simulink model "basic"  (R2018a)
settings: Solver=FixedStepAuto  StartTime=0.0  StopTime=inf  FixedStep=0.005  RelTol=1e-3  EnableMultiTasking=on
libraries: arduinolib x3, simulink x3
settings Model: SimulationMode=external  ExtModeTrigDuration=2  Creator=adiravishankara  LastModifiedBy=adiravishankara
settings SolverCC: AutoInsertRateTranBlk=on
settings OptimizationCC: EnhancedBackFolding=on  PassReuseOutputArgsAs=Individual arguments  MaxStackSize=64  OptimizeBlockOrder=speed  DifferentSizesBufferReuse=on  OptimizationCustomize=off
settings DebuggingCC: ParameterTunabilityLossMsg=error
settings HardwareCC: ProdBitPerPointer=32  ProdBitPerSizeT=32  ProdBitPerPtrDiffT=32  ProdLargestAtomicInteger=Long  ProdLargestAtomicFloat=Double  ProdWordSize=32  ProdHWDeviceType=ARM Compatible->ARM Cortex  UseEmbeddedCoderFeatures=off
settings SFSimCC: MATLABDynamicMemAlloc=off
settings RTWCC: SystemTargetFile=ert.tlc  HardwareBoard=Arduino Due  TLCOptions=-aInlineSetEventsForThisBaseRateFcn=TLC_FALSE -aSuppressMultiTaskScheduler=TLC_FALSE -aRateBasedStepFcn=1  TemplateMakefile=ert_default_tmf  GenerateReport=on  Toolchain=Arduino ARM  BuildConfiguration=Faster Runs  IncludeHyperlinkInReport=on  LaunchReport=on  GenerateTraceInfo=on  GenerateTraceReport=on  GenerateTraceReportSl=on  GenerateTraceReportSf=on  GenerateTraceReportEml=on
settings CodeAppCC: ForceParamTrailComments=on  IgnoreCustomStorageClasses=off  OperatorAnnotations=on  SimulinkDataObjDesc=on  SFDataObjDesc=on  InsertBlockDesc=on
settings ERTTargetCC: SupportContinuousTime=on  SupportNonInlinedSFcns=on  SupportVariableSizeSignals=on

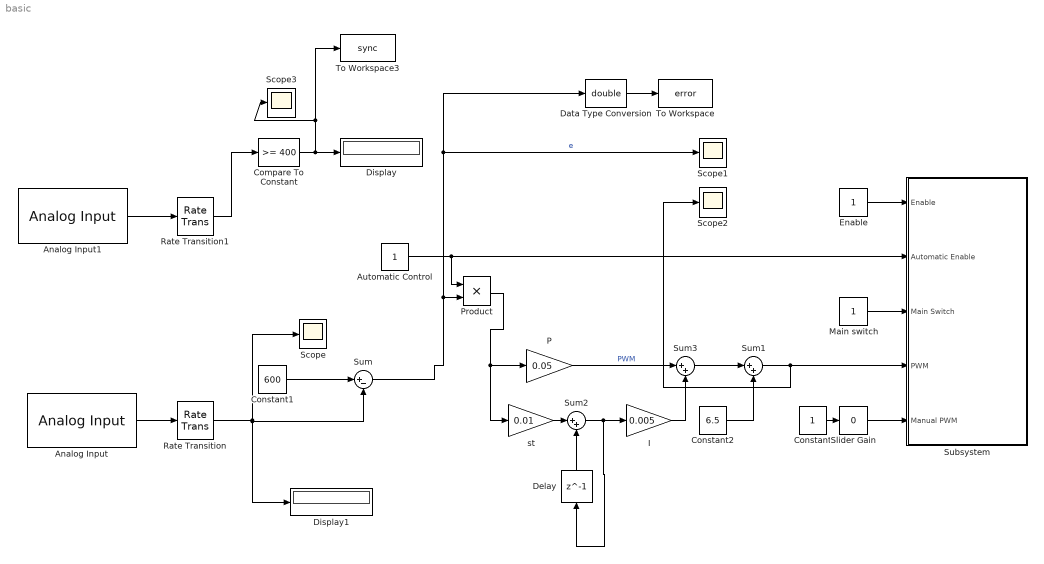
== system basic ==
  Analog Input : arduinolib/Analog Input  pinNumber=2  ReadResultsOnly=off  ConversionTriggerSource=Software  ExternalTriggerType=uint32(0)  OutputDataType=uint16  EnableConversionCompleteNotify=off  EnableOuputStatus=off  SampleTime=0.01  blockPlatform=arduino
  Analog Input1 : arduinolib/Analog Input  pinNumber=3  ReadResultsOnly=off  ConversionTriggerSource=Software  ExternalTriggerType=uint32(0)  OutputDataType=uint16  EnableConversionCompleteNotify=off  EnableOuputStatus=off  SampleTime=0.01  blockPlatform=arduino
  Automatic Control : Constant  SampleTime=0.01
  Compare To Constant : simulink/Logic and Bit Operations/Compare To Constant  relop=>=  const=400  OutDataTypeStr=boolean
  Constant : Constant  SampleTime=0.01
  Constant1 : Constant  Value=600  SampleTime=0.01
  Constant2 : Constant  Value=6.5  SampleTime=0.01
  Data Type Conversion : DataTypeConversion  OutDataTypeStr=double
  Delay : Delay  DelayLength=1  SampleTime=0.01
  Display : Display
  Display1 : Display
  Enable : Constant  SampleTime=0.01
  I : Gain  Gain=0.005
  Main switch : Constant  SampleTime=0.01
  P : Gain  Gain=0.05
  Product : Product
  Rate Transition : RateTransition  OutPortSampleTime=0.01
  Rate Transition1 : RateTransition  OutPortSampleTime=0.01
  Scope{,1..3} (4 alike) : Scope
  Slider Gain : simulink/Math Operations/Slider Gain  gain=0  low=0  high=40
  Subsystem : Subsystem
  Sum : Sum  Inputs=|+-
  Sum1 : Sum  Inputs=|++
  Sum2 : Sum  Inputs=|++
  Sum3 : Sum  Inputs=|++
  To Workspace : ToWorkspace  VariableName=error  SaveFormat=Structure With Time  SampleTime=-1
  To Workspace3 : ToWorkspace  VariableName=sync  SaveFormat=Timeseries  SampleTime=0.01
  st : Gain  Gain=0.01
  wires:
  P/1 -> Sum3/1  "PWM"
  Rate Transition1/1 -> Compare To Constant/1
  Analog Input1/1 -> Rate Transition1/1
  Sum3/1 -> Sum1/1
  Rate Transition/1 -> Display1/1, Sum/2, Scope/1
  I/1 -> Sum3/2
  Slider Gain/1 -> Subsystem/5(Manual PWM)
  Sum/1 -> Data Type Conversion/1, Scope1/1, Product/2  "e"
  Main switch/1 -> Subsystem/3(Main Switch)
  Product/1 -> st/1, P/1
  Automatic Control/1 -> Product/1, Subsystem/2(Automatic Enable)
  Sum1/1 -> Scope2/1, Subsystem/4(PWM)
  Delay/1 -> Sum2/2
  Sum2/1 -> Delay/1, I/1
  Constant2/1 -> Sum1/2
  st/1 -> Sum2/1
  Enable/1 -> Subsystem/1(Enable)
  Constant1/1 -> Sum/1
  Constant/1 -> Slider Gain/1
  Analog Input/1 -> Rate Transition/1
  Compare To Constant/1 -> Scope3/1, To Workspace3/1, Display/1
  Data Type Conversion/1 -> To Workspace/1

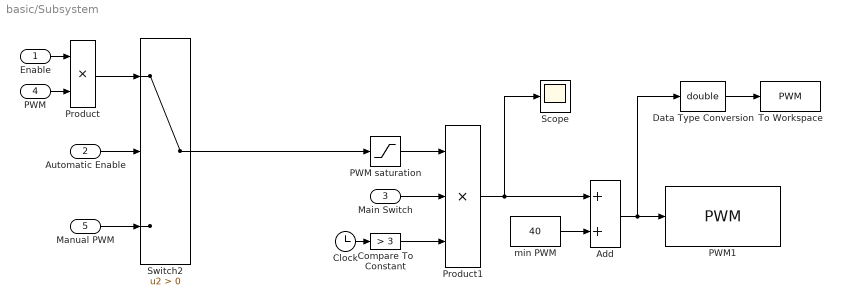
== system basic/Subsystem ==
  Enable : Inport
  Automatic Enable : Inport  Port=2
  Main Switch : Inport  Port=3
  PWM : Inport  Port=4
  Manual PWM : Inport  Port=5
  Add : Sum
  Clock : Clock
  Compare To Constant : simulink/Logic and Bit Operations/Compare To Constant  relop=>  const=3  OutDataTypeStr=boolean
  Data Type Conversion : DataTypeConversion  OutDataTypeStr=double
  PWM saturation : Saturate  UpperLimit=40  LowerLimit=0
  PWM1 : arduinolib/PWM  pinNumber=12  EnableInputFrequency=off  InitialFrequency=2000  InitialDutyCycle=0  NotificationType=None  blockPlatform=arduino
  Product : Product
  Product1 : Product  Inputs=3
  Scope : Scope
  Switch2 : Switch  Criteria=u2 > Threshold
  To Workspace : ToWorkspace  VariableName=PWM  SaveFormat=Structure With Time  SampleTime=-1
  min PWM : Constant  Value=40  SampleTime=0.01
  wires:
  Clock/1 -> Compare To Constant/1
  min PWM/1 -> Add/2
  Compare To Constant/1 -> Product1/3
  Automatic Enable/1 -> Switch2/2
  Add/1 -> PWM1/1, Data Type Conversion/1
  Manual PWM/1 -> Switch2/3
  PWM/1 -> Product/2
  Switch2/1 -> PWM saturation/1
  Main Switch/1 -> Product1/2
  Product1/1 -> Scope/1, Add/1
  PWM saturation/1 -> Product1/1
  Data Type Conversion/1 -> To Workspace/1
  Product/1 -> Switch2/1
  Enable/1 -> Product/1
